simulink model "Simulink_Model"  (R2022a)
settings: Solver=ode4  StartTime=0.0  StopTime=10  FixedStep=0.01  RelTol=1e-3
settings Model: Creator=nahiz  LastModifiedBy=nahiz

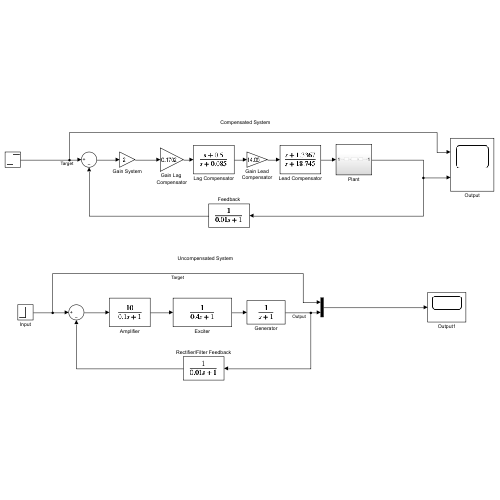
[thumbnail: Simulink's stored preview of the top-level diagram]
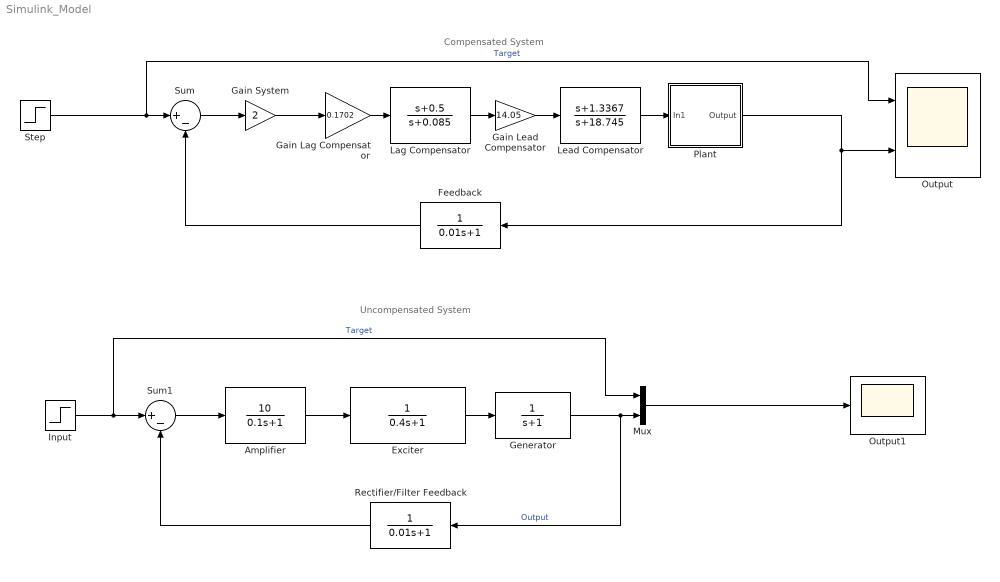
== system Simulink_Model ==
  note: Uncompensated System
  note: Compensated System
  Amplifier : TransferFcn  Numerator=[10]  Denominator=[0.1 1]
  Exciter : TransferFcn  Denominator=[0.4 1]
  Feedback : TransferFcn  Denominator=[0.01 1]
  Gain Lag Compensator : Gain  Gain=0.1702
  Gain Lead Compensator : Gain  Gain=14.05
  Gain System : Gain  Gain=2
  Generator : TransferFcn  Denominator=[1 1]
  Input : Step  Time=0  SampleTime=0.01
  Lag Compensator : TransferFcn  Numerator=[1 0.5]  Denominator=[1 0.085]
  Lead Compensator : TransferFcn  Numerator=[1 1.3367]  Denominator=[1 18.745]
  Mux : Mux  Inputs=2
  Output : Scope  NumInputPorts=2
  Output1 : Scope
  Plant : Subsystem
  Rectifier/Filter Feedback : TransferFcn  Denominator=[0.01 1]
  Step : Step  SampleTime=0
  Sum : Sum  Inputs=|+-
  Sum1 : Sum  Inputs=|+-
  wires:
  Feedback/1 -> Sum/2
  Plant/1(Output) -> Feedback/1, Output/2
  Lag Compensator/1 -> Gain Lead Compensator/1
  Gain System/1 -> Gain Lag Compensator/1
  Gain Lag Compensator/1 -> Lag Compensator/1
  Gain Lead Compensator/1 -> Lead Compensator/1
  Step/1 -> Output/1, Sum/1  "Target"
  Lead Compensator/1 -> Plant/1(In1)
  Sum/1 -> Gain System/1
  Mux/1 -> Output1/1
  Amplifier/1 -> Exciter/1
  Sum1/1 -> Amplifier/1
  Generator/1 -> Mux/2, Rectifier/Filter Feedback/1  "Output"
  Exciter/1 -> Generator/1
  Input/1 -> Mux/1, Sum1/1  "Target"
  Rectifier/Filter Feedback/1 -> Sum1/2

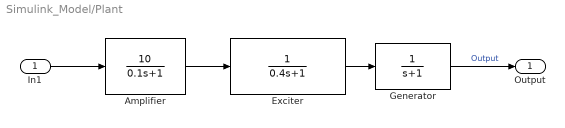
== system Simulink_Model/Plant ==
  In1 : Inport
  Amplifier : TransferFcn  Numerator=[10]  Denominator=[0.1 1]
  Exciter : TransferFcn  Denominator=[0.4 1]
  Generator : TransferFcn  Denominator=[1 1]
  Output : Outport
  wires:
  Generator/1 -> Output/1  "Output"
  Exciter/1 -> Generator/1
  Amplifier/1 -> Exciter/1
  In1/1 -> Amplifier/1
